simulink model "model"  (R2015b)
settings: Solver=VariableStepAuto  StartTime=0.0  StopTime=50  RelTol=1e-3
settings Model: Creator=Asus  LastModifiedBy=Asus

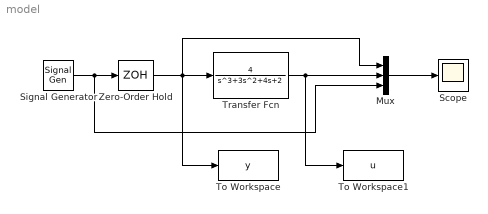
== system model ==
  Mux : Mux  Inputs=3
  Scope : Scope
  Signal Generator : SignalGenerator  Units=rad/sec
  To Workspace : ToWorkspace  VariableName=y  SampleTime=-1
  To Workspace1 : ToWorkspace  VariableName=u  SampleTime=-1
  Transfer Fcn : TransferFcn  Numerator=[4]  Denominator=[1 3 4 2]
  Zero-Order Hold : ZeroOrderHold
  wires:
  Signal Generator/1 -> Mux/3, Zero-Order Hold/1
  Zero-Order Hold/1 -> Mux/1, To Workspace/1, Transfer Fcn/1
  Transfer Fcn/1 -> To Workspace1/1, Mux/2
  Mux/1 -> Scope/1
